simulink model "SimpleUnitTC_SoftwareArch_WCC_mapping"  (R2016b)
settings: Solver=FixedStepAuto  StartTime=0.0  StopTime=10.0  RelTol=1e-3
model workspace: external: MAT-File SimpleUnitTC_SoftwareArch_WCC_mapping.mat (data not in the file)
libraries: libTLAsserts x8, libAsserts x3
settings Model: Creator=takiy  LastModifiedBy=takiy

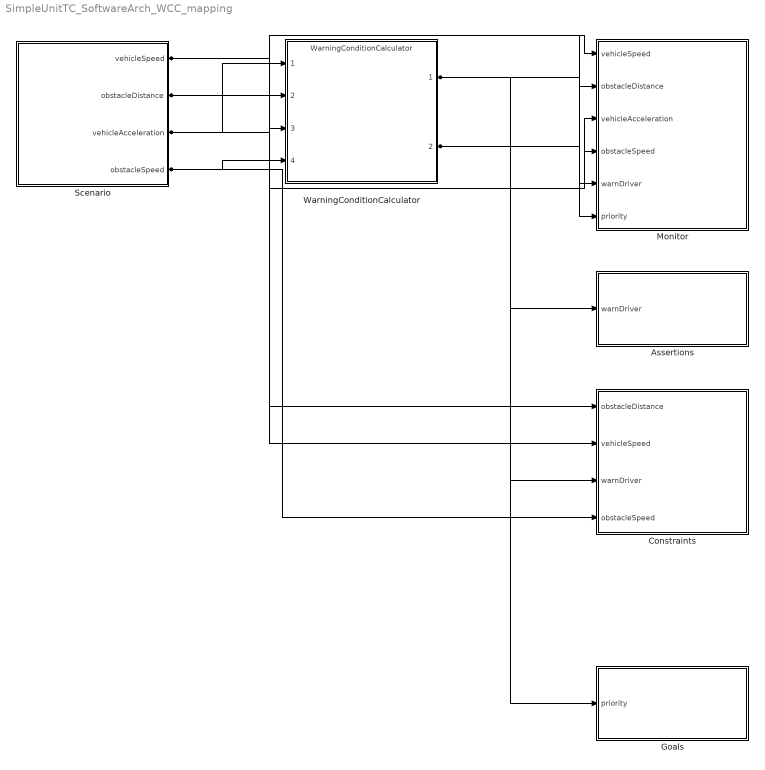
== system SimpleUnitTC_SoftwareArch_WCC_mapping ==
  Assertions : Subsystem
  Constraints : Subsystem
  Goals : Subsystem
  Monitor : Subsystem
  Scenario : Subsystem
  WarningConditionCalculator : ModelReference  ModelNameDialog=WarningConditionCalculator  SimulationMode=Normal  ModelReferenceVersion=1.9
  wires:
  Scenario/3(vehicleAcceleration) -> WarningConditionCalculator/1, Monitor/3(vehicleAcceleration)
  Scenario/1(vehicleSpeed) -> WarningConditionCalculator/2, Monitor/1(vehicleSpeed), Constraints/2(vehicleSpeed)
  Scenario/4(obstacleSpeed) -> WarningConditionCalculator/4, Monitor/4(obstacleSpeed), Constraints/4(obstacleSpeed)
  Scenario/2(obstacleDistance) -> WarningConditionCalculator/3, Monitor/2(obstacleDistance), Constraints/1(obstacleDistance)
  WarningConditionCalculator/1 -> Monitor/5(warnDriver), Assertions/1(warnDriver), Constraints/3(warnDriver)
  WarningConditionCalculator/2 -> Monitor/6(priority), Goals/1(priority)

== system SimpleUnitTC_SoftwareArch_WCC_mapping/Assertions ==
  warnDriver : Inport
  assert_1 : Subsystem
  simout_1 : ToFile  Filename=assert_1.mat  MatrixName=assert_1  SaveFormat=Timeseries
  wires:
  warnDriver/1 -> assert_1/1(warnDriver)
  assert_1/1(assert_1_FAILED) -> simout_1/1

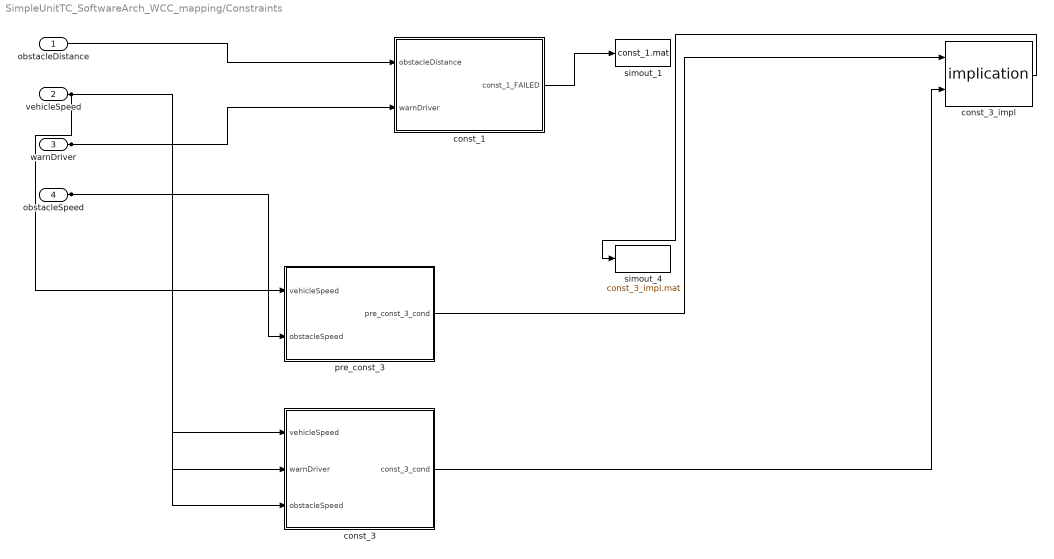
== system SimpleUnitTC_SoftwareArch_WCC_mapping/Constraints ==
  obstacleDistance : Inport
  vehicleSpeed : Inport  Port=2
  warnDriver : Inport  Port=3
  obstacleSpeed : Inport  Port=4
  const_1 : Subsystem
  const_3 : Subsystem
  const_3_impl : libAsserts/implication
  pre_const_3 : Subsystem
  simout_1 : ToFile  Filename=const_1.mat  MatrixName=const_1  SaveFormat=Timeseries
  simout_4 : ToFile  Filename=const_3_impl.mat  MatrixName=const_3_impl  SaveFormat=Timeseries
  wires:
  obstacleDistance/1 -> const_1/1(obstacleDistance)
  warnDriver/1 -> const_1/2(warnDriver), const_3/2(warnDriver)
  const_1/1(const_1_FAILED) -> simout_1/1
  vehicleSpeed/1 -> pre_const_3/1(vehicleSpeed), const_3/1(vehicleSpeed)
  obstacleSpeed/1 -> pre_const_3/2(obstacleSpeed), const_3/3(obstacleSpeed)
  pre_const_3/1(pre_const_3_cond) -> const_3_impl/1
  const_3/1(const_3_cond) -> const_3_impl/2
  const_3_impl/1 -> simout_4/1

== system SimpleUnitTC_SoftwareArch_WCC_mapping/Goals ==
  priority : Inport
  goals_1 : Subsystem
  simout_1 : ToFile  Filename=goals_1.mat  MatrixName=goals_1  SaveFormat=Timeseries
  wires:
  priority/1 -> goals_1/1(priority)
  goals_1/1(goals_1_VAL) -> simout_1/1

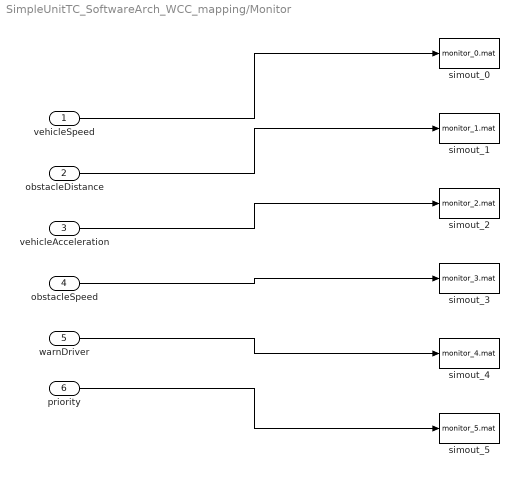
== system SimpleUnitTC_SoftwareArch_WCC_mapping/Monitor ==
  vehicleSpeed : Inport
  obstacleDistance : Inport  Port=2
  vehicleAcceleration : Inport  Port=3
  obstacleSpeed : Inport  Port=4
  warnDriver : Inport  Port=5
  priority : Inport  Port=6
  simout_0 : ToFile  Filename=monitor_0.mat  MatrixName=vehicleSpeed  SaveFormat=Timeseries
  simout_1 : ToFile  Filename=monitor_1.mat  MatrixName=obstacleDistance  SaveFormat=Timeseries
  simout_2 : ToFile  Filename=monitor_2.mat  MatrixName=vehicleAcceleration  SaveFormat=Timeseries
  simout_3 : ToFile  Filename=monitor_3.mat  MatrixName=obstacleSpeed  SaveFormat=Timeseries
  simout_4 : ToFile  Filename=monitor_4.mat  MatrixName=warnDriver  SaveFormat=Timeseries
  simout_5 : ToFile  Filename=monitor_5.mat  MatrixName=priority  SaveFormat=Timeseries
  wires:
  vehicleSpeed/1 -> simout_0/1
  obstacleDistance/1 -> simout_1/1
  vehicleAcceleration/1 -> simout_2/1
  obstacleSpeed/1 -> simout_3/1
  warnDriver/1 -> simout_4/1
  priority/1 -> simout_5/1

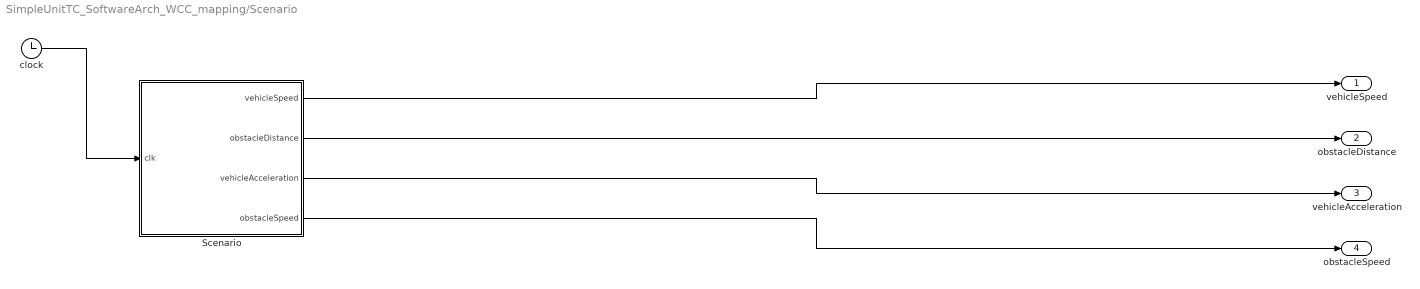
== system SimpleUnitTC_SoftwareArch_WCC_mapping/Scenario ==
  Scenario : Stateflow chart  TreatAsAtomicUnit=on
  clock : Clock
  vehicleSpeed : Outport
  obstacleDistance : Outport  Port=2
  vehicleAcceleration : Outport  Port=3
  obstacleSpeed : Outport  Port=4
  wires:
  Scenario/3(vehicleAcceleration) -> vehicleAcceleration/1
  Scenario/1(vehicleSpeed) -> vehicleSpeed/1
  Scenario/4(obstacleSpeed) -> obstacleSpeed/1
  Scenario/2(obstacleDistance) -> obstacleDistance/1
  clock/1 -> Scenario/1(clk)

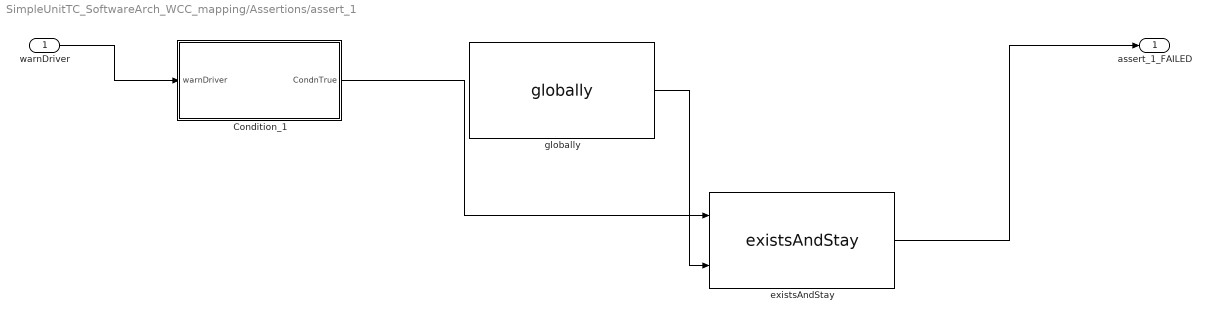
== system SimpleUnitTC_SoftwareArch_WCC_mapping/Assertions/assert_1 ==
  warnDriver : Inport
  Condition_1 : Subsystem
  existsAndStay : libTLAsserts/existsAndStay
  globally : libTLAsserts/globally
  assert_1_FAILED : Outport
  wires:
  warnDriver/1 -> Condition_1/1(warnDriver)
  Condition_1/1(CondnTrue) -> existsAndStay/1
  globally/1 -> existsAndStay/2
  existsAndStay/1 -> assert_1_FAILED/1

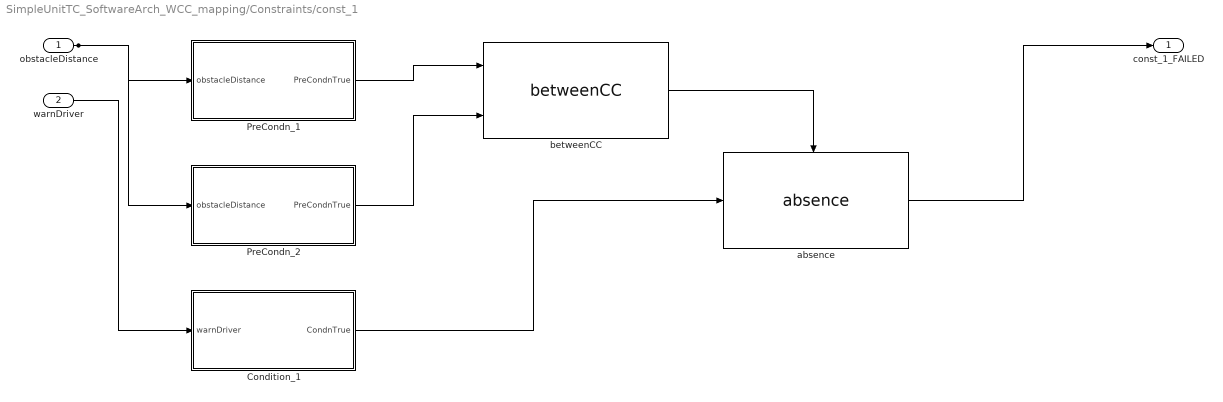
== system SimpleUnitTC_SoftwareArch_WCC_mapping/Constraints/const_1 ==
  obstacleDistance : Inport
  warnDriver : Inport  Port=2
  Condition_1 : Subsystem
  PreCondn_1 : Subsystem
  PreCondn_2 : Subsystem
  absence : libTLAsserts/absence
  betweenCC : libTLAsserts/betweenCC
  const_1_FAILED : Outport
  wires:
  obstacleDistance/1 -> PreCondn_1/1(obstacleDistance), PreCondn_2/1(obstacleDistance)
  warnDriver/1 -> Condition_1/1(warnDriver)
  PreCondn_1/1(PreCondnTrue) -> betweenCC/1
  PreCondn_2/1(PreCondnTrue) -> betweenCC/2
  Condition_1/1(CondnTrue) -> absence/1
  betweenCC/1 -> absence/Enable
  absence/1 -> const_1_FAILED/1

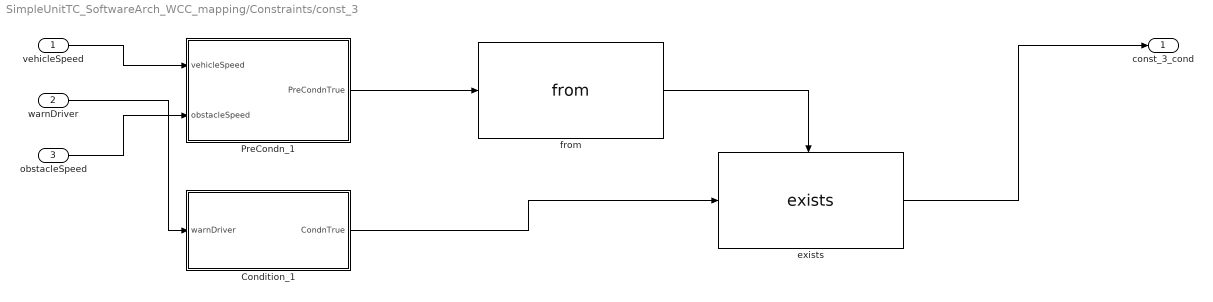
== system SimpleUnitTC_SoftwareArch_WCC_mapping/Constraints/const_3 ==
  vehicleSpeed : Inport
  warnDriver : Inport  Port=2
  obstacleSpeed : Inport  Port=3
  Condition_1 : Subsystem
  PreCondn_1 : Subsystem
  exists : libTLAsserts/exists
  from : libTLAsserts/from
  const_3_cond : Outport
  wires:
  vehicleSpeed/1 -> PreCondn_1/1(vehicleSpeed)
  obstacleSpeed/1 -> PreCondn_1/2(obstacleSpeed)
  warnDriver/1 -> Condition_1/1(warnDriver)
  PreCondn_1/1(PreCondnTrue) -> from/1
  Condition_1/1(CondnTrue) -> exists/1
  from/1 -> exists/Enable
  exists/1 -> const_3_cond/1

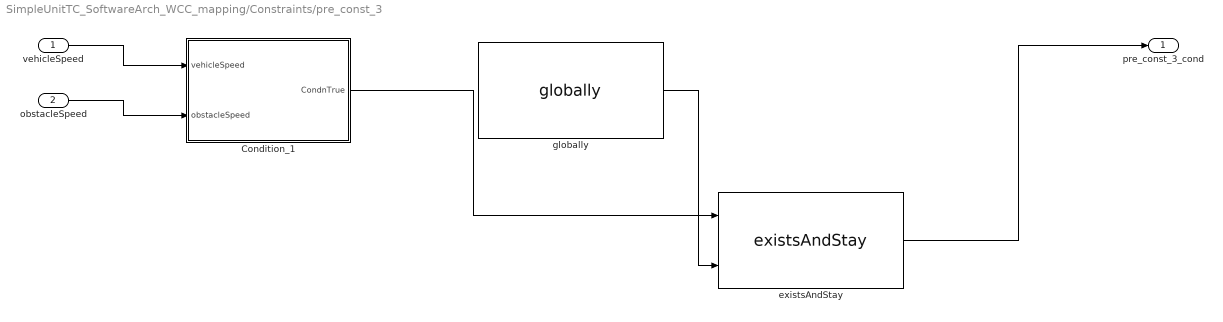
== system SimpleUnitTC_SoftwareArch_WCC_mapping/Constraints/pre_const_3 ==
  vehicleSpeed : Inport
  obstacleSpeed : Inport  Port=2
  Condition_1 : Subsystem
  existsAndStay : libTLAsserts/existsAndStay
  globally : libTLAsserts/globally
  pre_const_3_cond : Outport
  wires:
  vehicleSpeed/1 -> Condition_1/1(vehicleSpeed)
  obstacleSpeed/1 -> Condition_1/2(obstacleSpeed)
  Condition_1/1(CondnTrue) -> existsAndStay/1
  globally/1 -> existsAndStay/2
  existsAndStay/1 -> pre_const_3_cond/1

== system SimpleUnitTC_SoftwareArch_WCC_mapping/Goals/goals_1 ==
  priority : Inport
  goals_1_VAL : Outport
  wires:
  priority/1 -> goals_1_VAL/1

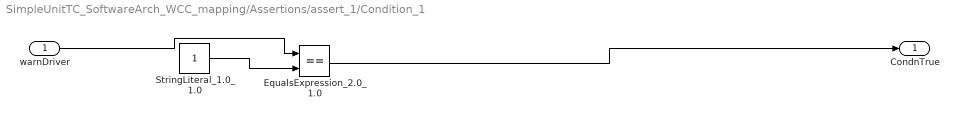
== system SimpleUnitTC_SoftwareArch_WCC_mapping/Assertions/assert_1/Condition_1 ==
  warnDriver : Inport
  EqualsExpression_2.0_1.0 : RelationalOperator  Operator===  OutDataTypeStr=boolean  RndMeth=Simplest
  StringLiteral_1.0_1.0 : Constant
  CondnTrue : Outport
  wires:
  warnDriver/1 -> EqualsExpression_2.0_1.0/1
  StringLiteral_1.0_1.0/1 -> EqualsExpression_2.0_1.0/2
  EqualsExpression_2.0_1.0/1 -> CondnTrue/1

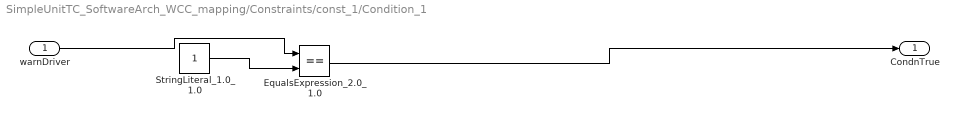
== system SimpleUnitTC_SoftwareArch_WCC_mapping/Constraints/const_1/Condition_1 ==
  warnDriver : Inport
  EqualsExpression_2.0_1.0 : RelationalOperator  Operator===  OutDataTypeStr=boolean  RndMeth=Simplest
  StringLiteral_1.0_1.0 : Constant
  CondnTrue : Outport
  wires:
  warnDriver/1 -> EqualsExpression_2.0_1.0/1
  StringLiteral_1.0_1.0/1 -> EqualsExpression_2.0_1.0/2
  EqualsExpression_2.0_1.0/1 -> CondnTrue/1

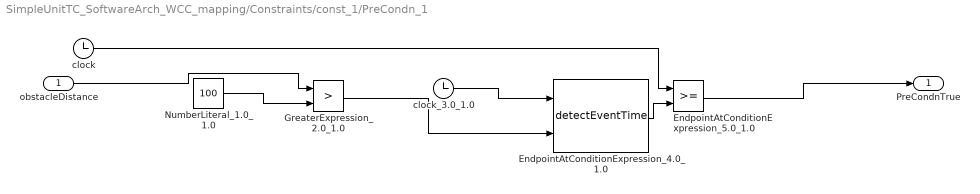
== system SimpleUnitTC_SoftwareArch_WCC_mapping/Constraints/const_1/PreCondn_1 ==
  obstacleDistance : Inport
  EndpointAtConditionExpression_4.0_1.0 : libAsserts/detectEventTime
  EndpointAtConditionExpression_5.0_1.0 : RelationalOperator  OutDataTypeStr=boolean  RndMeth=Simplest
  GreaterExpression_2.0_1.0 : RelationalOperator  Operator=>  OutDataTypeStr=boolean  RndMeth=Simplest
  NumberLiteral_1.0_1.0 : Constant  Value=100
  clock : Clock
  clock_3.0_1.0 : Clock
  PreCondnTrue : Outport
  wires:
  obstacleDistance/1 -> GreaterExpression_2.0_1.0/1
  NumberLiteral_1.0_1.0/1 -> GreaterExpression_2.0_1.0/2
  clock_3.0_1.0/1 -> EndpointAtConditionExpression_4.0_1.0/1
  GreaterExpression_2.0_1.0/1 -> EndpointAtConditionExpression_4.0_1.0/2
  clock/1 -> EndpointAtConditionExpression_5.0_1.0/1
  EndpointAtConditionExpression_4.0_1.0/1 -> EndpointAtConditionExpression_5.0_1.0/2
  EndpointAtConditionExpression_5.0_1.0/1 -> PreCondnTrue/1

== system SimpleUnitTC_SoftwareArch_WCC_mapping/Constraints/const_1/PreCondn_2 ==
  obstacleDistance : Inport
  LessExpression_2.0_1.0 : RelationalOperator  Operator=<  OutDataTypeStr=boolean  RndMeth=Simplest
  NumberLiteral_1.0_1.0 : Constant  Value=100
  PreCondnTrue : Outport
  wires:
  obstacleDistance/1 -> LessExpression_2.0_1.0/1
  NumberLiteral_1.0_1.0/1 -> LessExpression_2.0_1.0/2
  LessExpression_2.0_1.0/1 -> PreCondnTrue/1

== system SimpleUnitTC_SoftwareArch_WCC_mapping/Constraints/const_3/Condition_1 ==
  warnDriver : Inport
  EqualsExpression_2.0_1.0 : RelationalOperator  Operator===  OutDataTypeStr=boolean  RndMeth=Simplest
  StringLiteral_1.0_1.0 : Constant
  CondnTrue : Outport
  wires:
  warnDriver/1 -> EqualsExpression_2.0_1.0/1
  StringLiteral_1.0_1.0/1 -> EqualsExpression_2.0_1.0/2
  EqualsExpression_2.0_1.0/1 -> CondnTrue/1

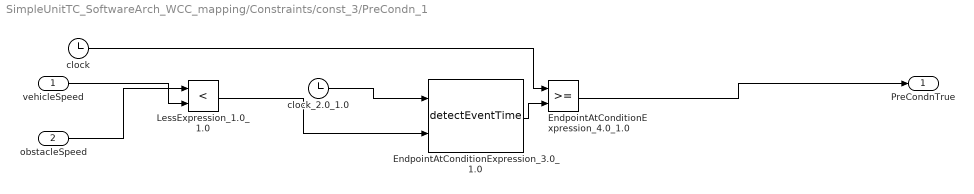
== system SimpleUnitTC_SoftwareArch_WCC_mapping/Constraints/const_3/PreCondn_1 ==
  vehicleSpeed : Inport
  obstacleSpeed : Inport  Port=2
  EndpointAtConditionExpression_3.0_1.0 : libAsserts/detectEventTime
  EndpointAtConditionExpression_4.0_1.0 : RelationalOperator  OutDataTypeStr=boolean  RndMeth=Simplest
  LessExpression_1.0_1.0 : RelationalOperator  Operator=<  OutDataTypeStr=boolean  RndMeth=Simplest
  clock : Clock
  clock_2.0_1.0 : Clock
  PreCondnTrue : Outport
  wires:
  obstacleSpeed/1 -> LessExpression_1.0_1.0/1
  vehicleSpeed/1 -> LessExpression_1.0_1.0/2
  clock_2.0_1.0/1 -> EndpointAtConditionExpression_3.0_1.0/1
  LessExpression_1.0_1.0/1 -> EndpointAtConditionExpression_3.0_1.0/2
  clock/1 -> EndpointAtConditionExpression_4.0_1.0/1
  EndpointAtConditionExpression_3.0_1.0/1 -> EndpointAtConditionExpression_4.0_1.0/2
  EndpointAtConditionExpression_4.0_1.0/1 -> PreCondnTrue/1

== system SimpleUnitTC_SoftwareArch_WCC_mapping/Constraints/pre_const_3/Condition_1 ==
  vehicleSpeed : Inport
  obstacleSpeed : Inport  Port=2
  LessExpression_1.0_1.0 : RelationalOperator  Operator=<  OutDataTypeStr=boolean  RndMeth=Simplest
  CondnTrue : Outport
  wires:
  obstacleSpeed/1 -> LessExpression_1.0_1.0/1
  vehicleSpeed/1 -> LessExpression_1.0_1.0/2
  LessExpression_1.0_1.0/1 -> CondnTrue/1

== stateflow chart SimpleUnitTC_SoftwareArch_WCC_mapping/Scenario/Scenario ==
  state Act_Subject [parallel]
    settings: executionOrder=1
    state Act_Subject_Step1
      entry: vehicleAcceleration = 0;
      entry: vehicleSpeed = 20;
      entry: Act_Subject_Step1_stpClk = clk;
    state Act_Subject_Step2
      entry: vehicleAcceleration = 1;
      entry: vehicleSpeed = vehicleSpeed + vehicleAcceleration * 1;
      entry: Act_Subject_Step2_stpClk = clk;
    state Act_Subject_Step3
    (default) -> Act_Subject_Step1
    Act_Subject_Step1 -> Act_Subject_Step2 : [clk - Act_Subject_Step1_stpClk > 1]
    Act_Subject_Step2 -> Act_Subject_Step3 : [clk - Act_Subject_Step2_stpClk > 1]
    Act_Subject_Step3 -> Act_Subject_Step2
  state Act_Obstacle [parallel]
    settings: executionOrder=2
    state Act_Obstacle_Step1
      entry: obstacleSpeed = vehicleSpeed;
      entry: obstacleDistance = 100;
    (default) -> Act_Obstacle_Step1
  data: clk input; vehicleSpeed output; obstacleDistance output; vehicleAcceleration output; obstacleSpeed output; Act_Subject_Step1_stpClk local; Act_Subject_Step2_stpClk local
